simulink model "hgo_diff_with_plant"  (R2024b)
settings: Solver=FixedStepAuto  StartTime=0.0  StopTime=15  FixedStep=1e-5  RelTol=1e-3
libraries: simulink x1
settings Model: Creator=user  LastModifiedBy=user

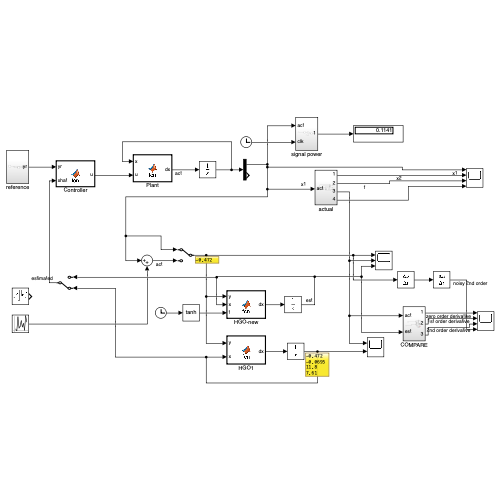
[thumbnail: Simulink's stored preview of the top-level diagram]
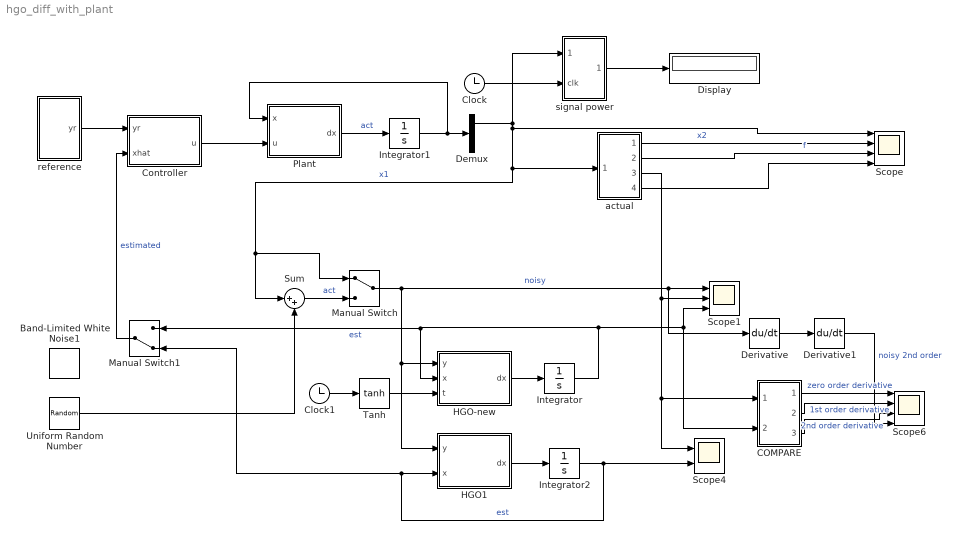
== system hgo_diff_with_plant ==
  Band-Limited White Noise1 : simulink/Sources/Band-Limited White Noise  Cov=1e-8  Ts=0.001  seed=[23341]
  COMPARE : Subsystem
  Clock : Clock
  Clock1 : Clock
  Controller : MATLAB Function  TreatAsAtomicUnit=on
  Demux : Demux  Outputs=[1 2]
  Derivative : Derivative
  Derivative1 : Derivative
  Display : Display
  HGO-new : MATLAB Function  TreatAsAtomicUnit=on
  HGO1 : MATLAB Function  TreatAsAtomicUnit=on
  Integrator : Integrator
  Integrator1 : Integrator
  Integrator2 : Integrator
  Manual Switch : ManualSwitch
  Manual Switch1 : ManualSwitch  CurrentSetting=0
  Plant : MATLAB Function  TreatAsAtomicUnit=on
  Scope : Scope  NumInputPorts=4
  Scope1 : Scope  NumInputPorts=3
  Scope4 : Scope  NumInputPorts=2
  Scope6 : Scope  NumInputPorts=4
  Sum : Sum  Inputs=|++
  Tanh : Trigonometry  Operator=tanh
  Uniform Random Number : UniformRandomNumber  Minimum=-1e-3  Maximum=1e-3  SampleTime=1e-3
  actual : Subsystem
  reference : Subsystem
  signal power : Subsystem
  wires:
  HGO-new/1(dx) -> Integrator/1
  Integrator/1 -> HGO-new/2(x), Manual Switch1/1, Scope1/3, COMPARE/2(est)  "est"
  Sum/1 -> Manual Switch/2  "act"
  Manual Switch/1 -> Scope1/1, Derivative/1, HGO-new/1(y), HGO1/1(y)  "noisy"
  HGO1/1(dx) -> Integrator2/1
  Integrator2/1 -> Scope4/2, Manual Switch1/2, HGO1/2(x)  "est"
  Clock/1 -> signal power/2(clk)
  COMPARE/1(Out1) -> Scope6/1  "zero order derivative"
  COMPARE/2(Out2) -> Scope6/2  "1st order derivative"
  COMPARE/3(Out3) -> Scope6/3  "2nd order derivative"
  actual/3(Out4) -> Scope1/2, COMPARE/1(act), Scope4/1
  actual/1(Out1) -> Scope/2  "x2"
  actual/2(Out2) -> Scope/3  "f"
  Derivative/1 -> Derivative1/1
  Derivative1/1 -> Scope6/4  "noisy 2nd order"
  Tanh/1 -> HGO-new/3(t)
  Uniform Random Number/1 -> Sum/2
  signal power/1(Out1) -> Display/1
  Integrator1/1 -> Plant/1(x), Demux/1
  Demux/1 -> Manual Switch/1, Sum/1, actual/1(act), Scope/1, signal power/1(act)  "x1"
  Clock1/1 -> Tanh/1
  Plant/1(dx) -> Integrator1/1  "act"
  Controller/1(u) -> Plant/2(u)
  reference/1(yr) -> Controller/1(yr)
  Manual Switch1/1 -> Controller/2(xhat)  "estimated"
  actual/4(Out3) -> Scope/4

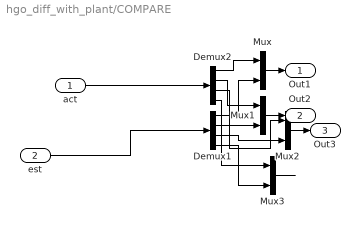
== system hgo_diff_with_plant/COMPARE ==
  act : Inport
  est : Inport  Port=2
  Demux1 : Demux
  Demux2 : Demux
  Mux{,1..3} (4 alike) : Mux  Inputs=2
  Out1 : Outport
  Out2 : Outport  Port=2
  Out3 : Outport  Port=3
  wires:
  est/1 -> Demux1/1
  Demux1/3 -> Mux2/2
  act/1 -> Demux2/1
  Demux2/1 -> Mux/1
  Mux3/1 -> ?
  Mux/1 -> Out1/1
  Demux1/2 -> Mux1/2
  Demux1/1 -> Mux/2
  Demux2/2 -> Mux1/1
  Mux2/1 -> Out3/1
  Demux2/3 -> Mux2/1
  Demux2/4 -> Mux3/1
  Mux1/1 -> Out2/1
  Demux1/4 -> Mux3/2

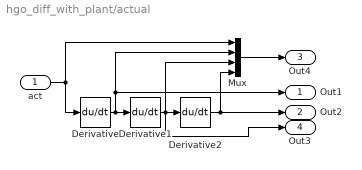
== system hgo_diff_with_plant/actual ==
  act : Inport
  Derivative : Derivative
  Derivative1 : Derivative
  Derivative2 : Derivative
  Mux : Mux
  Out1 : Outport
  Out2 : Outport  Port=2
  Out4 : Outport  Port=3
  Out3 : Outport  Port=4
  wires:
  Derivative/1 -> Out1/1, Mux/2, Derivative1/1
  act/1 -> Derivative/1, Mux/1
  Mux/1 -> Out4/1
  Derivative1/1 -> Out3/1, Derivative2/1, Mux/3
  Derivative2/1 -> Out2/1, Mux/4

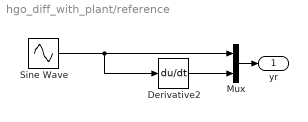
== system hgo_diff_with_plant/reference ==
  Derivative2 : Derivative
  Mux : Mux  Inputs=2
  Sine Wave : Sin  Frequency=5  SampleTime=0
  yr : Outport
  wires:
  Derivative2/1 -> Mux/2
  Sine Wave/1 -> Mux/1, Derivative2/1
  Mux/1 -> yr/1

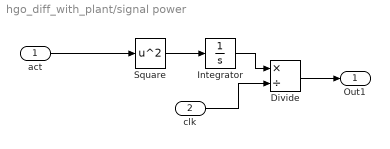
== system hgo_diff_with_plant/signal power ==
  act : Inport
  clk : Inport  Port=2
  Divide : Product  Inputs=*/
  Integrator : Integrator
  Square : Math  Operator=square
  Out1 : Outport
  wires:
  Square/1 -> Integrator/1
  act/1 -> Square/1
  Integrator/1 -> Divide/1
  clk/1 -> Divide/2
  Divide/1 -> Out1/1

== matlab function hgo_diff_with_plant/Controller ==
  data: yr input; u output; xhat input
function u = fcn(yr, xhat)
%e = error; de = e_dot
kp = 3; kd = 5;
e = yr - xhat(1:2);
u = kp*e(1) + kd*e(2)-xhat(3);

== matlab function hgo_diff_with_plant/Plant ==
  data: x input; dx output; u input
function dx = fcn(x, u)
% x = [x1; x2; f]

dx = zeros(3,1);
A = [0 1 0;
      0 0 1;
      0 0 0];
B = [0; 1; 0];
F = [0; 0; 1];
C = [1; 0; 0];

dx = A*x + B*u + F*x(3);

== matlab function hgo_diff_with_plant/HGO-new ==
  data: y input; dx output; x input; t input
function dx = fcn(y, x, t)
    % Parameters
    n = 4;                % Order of the observer
    epsilon = 1/200;      % Small gain parameter
    tr = t/10; 
    % Binomial coefficients (for n = 4)
    % ki = nchoosek(n, i)
    k = [4, 6, 4, 1]; 

    e = 1e-5;
    % Initialize output derivative
    dx = zeros(n, 1);
    
    % High-Gain Observer Equations
    dx(1) = x(2) + (k(1)*(tr+e)^1 / epsilon^1) * (y - x(1));
    dx(2) = x(3) + (k(2)*(tr+e)^2 / epsilon^2) * (y - x(1));
    dx(3) = x(4) + (k(3)*(tr+e)^3 / epsilon^3) * (y - x(1));
    dx(4) = (k(4)*(tr+e)^4 / epsilon^4) * (y - x(1));
end

== matlab function hgo_diff_with_plant/HGO1 ==
  data: y input; dx output; x input
function dx = fcn(y, x)
    % Parameters
    n = 4;                % Order of the observer
    epsilon = 1/200;      % Small gain parameter
    % tr = 1 ; 
    % Binomial coefficients (for n = 4)
    % ki = nchoosek(n, i)
    k = [4, 6, 4, 1]; 

    % Initialize output derivative
    dx = zeros(n, 1);
    
    % High-Gain Observer Equations
    dx(1) = x(2) + (k(1) / epsilon^1) * (y - x(1));
    dx(2) = x(3) + (k(2) / epsilon^2) * (y - x(1));
    dx(3) = x(4) + (k(3) / epsilon^3) * (y - x(1));
    dx(4) = (k(4) / epsilon^4) * (y - x(1));
end
